simulink model "intelligent_vehicle_example3"  (R2017a)
settings: Solver=VariableStepAuto  StartTime=0.0  StopTime=10.0  RelTol=1e-3
InitFcn:
  | c=1;
  | k=2;
  | m=5;
settings Model: Creator=edward  LastModifiedBy=edward

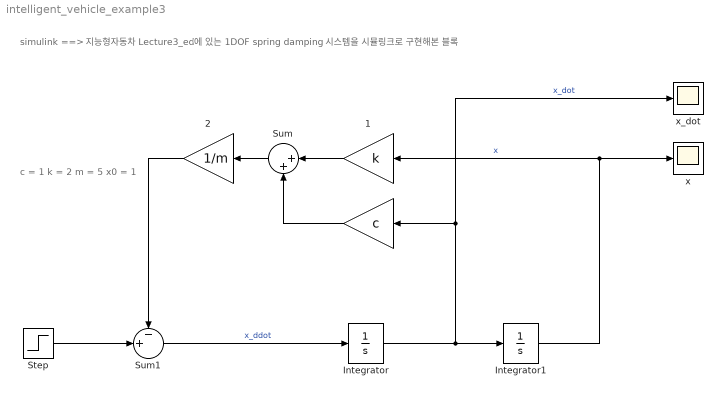
== system intelligent_vehicle_example3 ==
  note: c = 1
      | k = 2
      | m = 5
      | x0 = 1
  note: simulink ==> 지능형자동차 Lecture3_ed에 있는 1DOF spring damping 시스템을 시뮬링크로 구현해본 블록
  " " : Gain  Gain=c
  " 1" : Gain  Gain=k
  " 2" : Gain  Gain=1/m
  Integrator : Integrator
  Integrator1 : Integrator  InitialCondition=1
  Step : Step  Time=0  After=0  SampleTime=0
  Sum : Sum  Inputs=|++
  Sum1 : Sum  Inputs=-+|
  x : Scope
  x_dot : Scope
  wires:
  " 2"/1 -> Sum1/1
  Step/1 -> Sum1/2
  Integrator/1 -> x_dot/1, " "/1, Integrator1/1  "x_dot"
  " "/1 -> Sum/2
  Integrator1/1 -> " 1"/1, x/1  "x"
  Sum/1 -> " 2"/1
  Sum1/1 -> Integrator/1  "x_ddot"
  " 1"/1 -> Sum/1
